simulink model "problem4"  (R2020b)
settings: Solver=VariableStepAuto  StartTime=0.0  StopTime=30  MaxStep=0.01  RelTol=1e-3
settings Model: Creator=Varun  LastModifiedBy=Varun

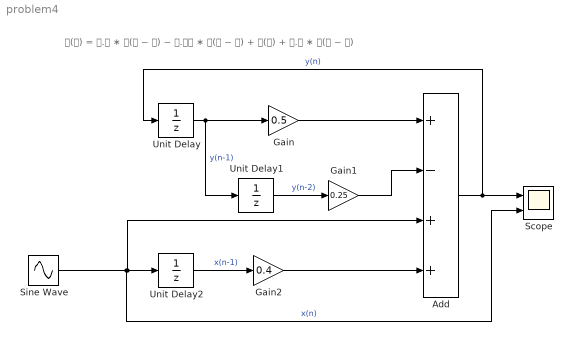
== system problem4 ==
  note: 𝐲(𝐧) = 𝟎.𝟓 ∗ 𝐲(𝐧 − 𝟏) − 𝟎.𝟐𝟓 ∗ 𝐲(𝐧 − 𝟐) + 𝐱(𝐧) + 𝟎.𝟒 ∗ 𝐱(𝐧 − 𝟏)
  Add : Sum  Inputs=+-++
  Gain : Gain  Gain=0.5
  Gain1 : Gain  Gain=0.25
  Gain2 : Gain  Gain=0.4
  Scope : Scope  NumInputPorts=2
  Sine Wave : Sin  SampleTime=0
  Unit Delay : UnitDelay  SampleTime=-1  HasFrameUpgradeWarning=on
  Unit Delay1 : UnitDelay  SampleTime=-1  HasFrameUpgradeWarning=on
  Unit Delay2 : UnitDelay  SampleTime=-1  HasFrameUpgradeWarning=on
  wires:
  Unit Delay/1 -> Unit Delay1/1, Gain/1  "y(n-1)"
  Unit Delay1/1 -> Gain1/1  "y(n-2)"
  Unit Delay2/1 -> Gain2/1  "x(n-1)"
  Add/1 -> Scope/1, Unit Delay/1  "y(n)"
  Sine Wave/1 -> Scope/2, Add/3, Unit Delay2/1  "x(n)"
  Gain/1 -> Add/1
  Gain2/1 -> Add/4
  Gain1/1 -> Add/2
